simulink model "MPC_stateflow"  (R2018b)
settings: Solver=ode4  StartTime=0.0  StopTime=10  FixedStep=0.05  RelTol=1e-3
libraries: neural x102
(part 3 of 3)

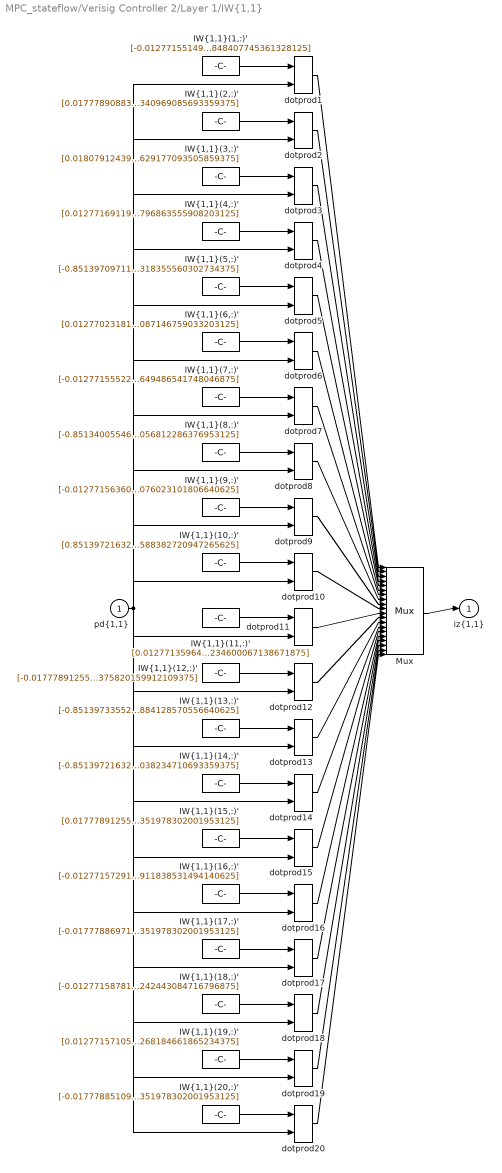
== system MPC_stateflow/Verisig Controller 2/Layer 1/IW{1,1} ==
  "pd{1,1}" : Inport  PortDimensions=6
      mask Display: e = 0.06;c1 = [120 230 180]/255;c2 = ([120 230 180]+0)/(256+128);c3 = ([120 230 180]+128)/(256+128);patch([0 1 1 0],[0 0 1 1],c1);patch([0 1 1 1-e 1-e 0+e],[0 0 1 1-e 0+e 0+e],c2);patch([0 0 1 1-e 0+e 0+e],[0 1 1 1-e 1-e 0+e],c3);plot([0 1 1 0 0],[0 0 1 1 0]);
  "IW{1,1}(1,:)'" : Constant  Value=[-0.012771551497280597686767578125;0.85226726531982421875;0.005031325854361057281494140625;0.0104131400585174560546875;0.52280867099761962890625;0.0038109351880848407745361328125]
      mask Display: e = 0.06;c1 = [120 150 230]/255;c2 = ([120 150 230]+0)/383;c3 = ([120 150 230]+128)/383;patch([0 1 1 0],[0 0 1 1],c1);patch([0 1 1 1-e 1-e 0+e],[0 0 1 1-e 0+e 0+e],c2);patch([0 0 1 1-e 0+e 0+e],[0 1 1 1-e 1-e 0+e],c3);plot([0 1 1 0 0],[0 0 1 1 0]);disp('Weights');
  "IW{1,1}(10,:)'" : Constant  Value=[0.851397216320037841796875;0.016397155821323394775390625;0.01527906768023967742919921875;0.523764669895172119140625;0.0148618109524250030517578125;0.008371211588382720947265625]
      mask Display: e = 0.06;c1 = [120 150 230]/255;c2 = ([120 150 230]+0)/383;c3 = ([120 150 230]+128)/383;patch([0 1 1 0],[0 0 1 1],c1);patch([0 1 1 1-e 1-e 0+e],[0 0 1 1-e 0+e 0+e],c2);patch([0 0 1 1-e 0+e 0+e],[0 1 1 1-e 1-e 0+e],c3);plot([0 1 1 0 0],[0 0 1 1 0]);disp('Weights');
  "IW{1,1}(11,:)'" : Constant  Value=[0.012771359644830226898193359375;-0.85226726531982421875;-0.0050320657901465892791748046875;-0.01041328720748424530029296875;-0.52280867099761962890625;-0.00381127069704234600067138671875]
      mask Display: e = 0.06;c1 = [120 150 230]/255;c2 = ([120 150 230]+0)/383;c3 = ([120 150 230]+128)/383;patch([0 1 1 0],[0 0 1 1],c1);patch([0 1 1 1-e 1-e 0+e],[0 0 1 1-e 0+e 0+e],c2);patch([0 0 1 1-e 0+e 0+e],[0 1 1 1-e 1-e 0+e],c3);plot([0 1 1 0 0],[0 0 1 1 0]);disp('Weights');
  "IW{1,1}(12,:)'" : Constant  Value=[-0.01777891255915164947509765625;-0.011899505741894245147705078125;0.8380184173583984375;-0.010888525284826755523681640625;-0.011424724943935871124267578125;0.54499375820159912109375]
      mask Display: e = 0.06;c1 = [120 150 230]/255;c2 = ([120 150 230]+0)/383;c3 = ([120 150 230]+128)/383;patch([0 1 1 0],[0 0 1 1],c1);patch([0 1 1 1-e 1-e 0+e],[0 0 1 1-e 0+e 0+e],c2);patch([0 0 1 1-e 0+e 0+e],[0 1 1 1-e 1-e 0+e],c3);plot([0 1 1 0 0],[0 0 1 1 0]);disp('Weights');
  "IW{1,1}(13,:)'" : Constant  Value=[-0.851397335529327392578125;-0.01639718003571033477783203125;-0.01527908630669116973876953125;-0.5237643718719482421875;-0.014861813746392726898193359375;-0.00837124884128570556640625]
      mask Display: e = 0.06;c1 = [120 150 230]/255;c2 = ([120 150 230]+0)/383;c3 = ([120 150 230]+128)/383;patch([0 1 1 0],[0 0 1 1],c1);patch([0 1 1 1-e 1-e 0+e],[0 0 1 1-e 0+e 0+e],c2);patch([0 0 1 1-e 0+e 0+e],[0 1 1 1-e 1-e 0+e],c3);plot([0 1 1 0 0],[0 0 1 1 0]);disp('Weights');
  "IW{1,1}(14,:)'" : Constant  Value=[-0.851397216320037841796875;-0.01639718748629093170166015625;-0.015279074199497699737548828125;-0.523764550685882568359375;-0.014861782081425189971923828125;-0.00837126933038234710693359375]
      mask Display: e = 0.06;c1 = [120 150 230]/255;c2 = ([120 150 230]+0)/383;c3 = ([120 150 230]+128)/383;patch([0 1 1 0],[0 0 1 1],c1);patch([0 1 1 1-e 1-e 0+e],[0 0 1 1-e 0+e 0+e],c2);patch([0 0 1 1-e 0+e 0+e],[0 1 1 1-e 1-e 0+e],c3);plot([0 1 1 0 0],[0 0 1 1 0]);disp('Weights');
  "IW{1,1}(15,:)'" : Constant  Value=[0.01777891255915164947509765625;0.011899520643055438995361328125;-0.838018596172332763671875;0.010888495482504367828369140625;0.0114247240126132965087890625;-0.54499351978302001953125]
      mask Display: e = 0.06;c1 = [120 150 230]/255;c2 = ([120 150 230]+0)/383;c3 = ([120 150 230]+128)/383;patch([0 1 1 0],[0 0 1 1],c1);patch([0 1 1 1-e 1-e 0+e],[0 0 1 1-e 0+e 0+e],c2);patch([0 0 1 1-e 0+e 0+e],[0 1 1 1-e 1-e 0+e],c3);plot([0 1 1 0 0],[0 0 1 1 0]);disp('Weights');
  "IW{1,1}(16,:)'" : Constant  Value=[-0.0127715729176998138427734375;0.85226726531982421875;0.0050313179381191730499267578125;0.010413181968033313751220703125;0.52280867099761962890625;0.0038109519518911838531494140625]
      mask Display: e = 0.06;c1 = [120 150 230]/255;c2 = ([120 150 230]+0)/383;c3 = ([120 150 230]+128)/383;patch([0 1 1 0],[0 0 1 1],c1);patch([0 1 1 1-e 1-e 0+e],[0 0 1 1-e 0+e 0+e],c2);patch([0 0 1 1-e 0+e 0+e],[0 1 1 1-e 1-e 0+e],c3);plot([0 1 1 0 0],[0 0 1 1 0]);disp('Weights');
  "IW{1,1}(17,:)'" : Constant  Value=[-0.0177788697183132171630859375;-0.01189949549734592437744140625;0.83801853656768798828125;-0.010888428427278995513916015625;-0.011424727737903594970703125;0.54499351978302001953125]
      mask Display: e = 0.06;c1 = [120 150 230]/255;c2 = ([120 150 230]+0)/383;c3 = ([120 150 230]+128)/383;patch([0 1 1 0],[0 0 1 1],c1);patch([0 1 1 1-e 1-e 0+e],[0 0 1 1-e 0+e 0+e],c2);patch([0 0 1 1-e 0+e 0+e],[0 1 1 1-e 1-e 0+e],c3);plot([0 1 1 0 0],[0 0 1 1 0]);disp('Weights');
  "IW{1,1}(18,:)'" : Constant  Value=[-0.0127715878188610076904296875;0.852267444133758544921875;0.0050312615931034088134765625;0.010413181968033313751220703125;0.52280843257904052734375;0.00381095963530242443084716796875]
      mask Display: e = 0.06;c1 = [120 150 230]/255;c2 = ([120 150 230]+0)/383;c3 = ([120 150 230]+128)/383;patch([0 1 1 0],[0 0 1 1],c1);patch([0 1 1 1-e 1-e 0+e],[0 0 1 1-e 0+e 0+e],c2);patch([0 0 1 1-e 0+e 0+e],[0 1 1 1-e 1-e 0+e],c3);plot([0 1 1 0 0],[0 0 1 1 0]);disp('Weights');
  "IW{1,1}(19,:)'" : Constant  Value=[0.01277157105505466461181640625;-0.852267205715179443359375;-0.005031269975006580352783203125;-0.0104131735861301422119140625;-0.522808611392974853515625;-0.0038109286688268184661865234375]
      mask Display: e = 0.06;c1 = [120 150 230]/255;c2 = ([120 150 230]+0)/383;c3 = ([120 150 230]+128)/383;patch([0 1 1 0],[0 0 1 1],c1);patch([0 1 1 1-e 1-e 0+e],[0 0 1 1-e 0+e 0+e],c2);patch([0 0 1 1-e 0+e 0+e],[0 1 1 1-e 1-e 0+e],c3);plot([0 1 1 0 0],[0 0 1 1 0]);disp('Weights');
  "IW{1,1}(2,:)'" : Constant  Value=[0.01777890883386135101318359375;0.011899493634700775146484375;-0.838018715381622314453125;0.01088852994143962860107421875;0.011424682103097438812255859375;-0.544993340969085693359375]
      mask Display: e = 0.06;c1 = [120 150 230]/255;c2 = ([120 150 230]+0)/383;c3 = ([120 150 230]+128)/383;patch([0 1 1 0],[0 0 1 1],c1);patch([0 1 1 1-e 1-e 0+e],[0 0 1 1-e 0+e 0+e],c2);patch([0 0 1 1-e 0+e 0+e],[0 1 1 1-e 1-e 0+e],c3);plot([0 1 1 0 0],[0 0 1 1 0]);disp('Weights');
  "IW{1,1}(20,:)'" : Constant  Value=[-0.017778851091861724853515625;-0.011899485252797603607177734375;0.83801853656768798828125;-0.010888493619859218597412109375;-0.0114247165620326995849609375;0.54499351978302001953125]
      mask Display: e = 0.06;c1 = [120 150 230]/255;c2 = ([120 150 230]+0)/383;c3 = ([120 150 230]+128)/383;patch([0 1 1 0],[0 0 1 1],c1);patch([0 1 1 1-e 1-e 0+e],[0 0 1 1-e 0+e 0+e],c2);patch([0 0 1 1-e 0+e 0+e],[0 1 1 1-e 1-e 0+e],c3);plot([0 1 1 0 0],[0 0 1 1 0]);disp('Weights');
  "IW{1,1}(3,:)'" : Constant  Value=[0.018079124391078948974609375;0.012226282618939876556396484375;-0.8379306793212890625;0.011077952571213245391845703125;0.011494635604321956634521484375;-0.54510629177093505859375]
      mask Display: e = 0.06;c1 = [120 150 230]/255;c2 = ([120 150 230]+0)/383;c3 = ([120 150 230]+128)/383;patch([0 1 1 0],[0 0 1 1],c1);patch([0 1 1 1-e 1-e 0+e],[0 0 1 1-e 0+e 0+e],c2);patch([0 0 1 1-e 0+e 0+e],[0 1 1 1-e 1-e 0+e],c3);plot([0 1 1 0 0],[0 0 1 1 0]);disp('Weights');
  "IW{1,1}(4,:)'" : Constant  Value=[0.012771691195666790008544921875;-0.852267205715179443359375;-0.005030765198171138763427734375;-0.010413102805614471435546875;-0.5228087902069091796875;-0.00381070119328796863555908203125]
      mask Display: e = 0.06;c1 = [120 150 230]/255;c2 = ([120 150 230]+0)/383;c3 = ([120 150 230]+128)/383;patch([0 1 1 0],[0 0 1 1],c1);patch([0 1 1 1-e 1-e 0+e],[0 0 1 1-e 0+e 0+e],c2);patch([0 0 1 1-e 0+e 0+e],[0 1 1 1-e 1-e 0+e],c3);plot([0 1 1 0 0],[0 0 1 1 0]);disp('Weights');
  "IW{1,1}(5,:)'" : Constant  Value=[-0.851397097110748291015625;-0.01639718748629093170166015625;-0.015279111452400684356689453125;-0.52376461029052734375;-0.014861795119941234588623046875;-0.008371188305318355560302734375]
      mask Display: e = 0.06;c1 = [120 150 230]/255;c2 = ([120 150 230]+0)/383;c3 = ([120 150 230]+128)/383;patch([0 1 1 0],[0 0 1 1],c1);patch([0 1 1 1-e 1-e 0+e],[0 0 1 1-e 0+e 0+e],c2);patch([0 0 1 1-e 0+e 0+e],[0 1 1 1-e 1-e 0+e],c3);plot([0 1 1 0 0],[0 0 1 1 0]);disp('Weights');
  "IW{1,1}(6,:)'" : Constant  Value=[0.0127702318131923675537109375;-0.852267563343048095703125;-0.0050366655923426151275634765625;-0.010414107702672481536865234375;-0.522808074951171875;-0.003813070245087146759033203125]
      mask Display: e = 0.06;c1 = [120 150 230]/255;c2 = ([120 150 230]+0)/383;c3 = ([120 150 230]+128)/383;patch([0 1 1 0],[0 0 1 1],c1);patch([0 1 1 1-e 1-e 0+e],[0 0 1 1-e 0+e 0+e],c2);patch([0 0 1 1-e 0+e 0+e],[0 1 1 1-e 1-e 0+e],c3);plot([0 1 1 0 0],[0 0 1 1 0]);disp('Weights');
  "IW{1,1}(7,:)'" : Constant  Value=[-0.012771555222570896148681640625;0.85226726531982421875;0.0050313002429902553558349609375;0.01041315495967864990234375;0.52280867099761962890625;0.003810915164649486541748046875]
      mask Display: e = 0.06;c1 = [120 150 230]/255;c2 = ([120 150 230]+0)/383;c3 = ([120 150 230]+128)/383;patch([0 1 1 0],[0 0 1 1],c1);patch([0 1 1 1-e 1-e 0+e],[0 0 1 1-e 0+e 0+e],c2);patch([0 0 1 1-e 0+e 0+e],[0 1 1 1-e 1-e 0+e],c3);plot([0 1 1 0 0],[0 0 1 1 0]);disp('Weights');
  "IW{1,1}(8,:)'" : Constant  Value=[-0.8513400554656982421875;-0.017523847520351409912109375;-0.01597718894481658935546875;-0.523753225803375244140625;-0.015967547893524169921875;-0.009223726578056812286376953125]
      mask Display: e = 0.06;c1 = [120 150 230]/255;c2 = ([120 150 230]+0)/383;c3 = ([120 150 230]+128)/383;patch([0 1 1 0],[0 0 1 1],c1);patch([0 1 1 1-e 1-e 0+e],[0 0 1 1-e 0+e 0+e],c2);patch([0 0 1 1-e 0+e 0+e],[0 1 1 1-e 1-e 0+e],c3);plot([0 1 1 0 0],[0 0 1 1 0]);disp('Weights');
  "IW{1,1}(9,:)'" : Constant  Value=[-0.01277156360447406768798828125;0.852267205715179443359375;0.0050313319079577922821044921875;0.010413155891001224517822265625;0.5228087902069091796875;0.0038109072484076023101806640625]
      mask Display: e = 0.06;c1 = [120 150 230]/255;c2 = ([120 150 230]+0)/383;c3 = ([120 150 230]+128)/383;patch([0 1 1 0],[0 0 1 1],c1);patch([0 1 1 1-e 1-e 0+e],[0 0 1 1-e 0+e 0+e],c2);patch([0 0 1 1-e 0+e 0+e],[0 1 1 1-e 1-e 0+e],c3);plot([0 1 1 0 0],[0 0 1 1 0]);disp('Weights');
  Mux : Mux  Inputs=20
      mask Display: e = 0.06;c1 = [120 150 230]/255;c2 = ([120 150 230]+0)/383;c3 = ([120 150 230]+128)/383;patch([0 1 1 0],[0 0 1 1],c1);patch([0 1 1 1-e 1-e 0+e],[0 0 1 1-e 0+e 0+e],c2);patch([0 0 1 1-e 0+e 0+e],[0 1 1 1-e 1-e 0+e],c3);plot([0 1 1 0 0],[0 0 1 1 0]);disp('Mux');
  dotprod{1..20} (20 alike) : neural/Weight Functions/dotprod
  "iz{1,1}" : Outport
      mask Display: e = 0.06;c1 = [120 230 180]/255;c2 = ([120 230 180]+0)/(256+128);c3 = ([120 230 180]+128)/(256+128);patch([0 1 1 0],[0 0 1 1],c1);patch([0 1 1 1-e 1-e 0+e],[0 0 1 1-e 0+e 0+e],c2);patch([0 0 1 1-e 0+e 0+e],[0 1 1 1-e 1-e 0+e],c3);plot([0 1 1 0 0],[0 0 1 1 0]);
  wires:
  Mux/1 -> "iz{1,1}"/1
  dotprod20/1 -> Mux/20
  "IW{1,1}(20,:)'"/1 -> dotprod20/1
  dotprod19/1 -> Mux/19
  "IW{1,1}(19,:)'"/1 -> dotprod19/1
  dotprod18/1 -> Mux/18
  "IW{1,1}(18,:)'"/1 -> dotprod18/1
  dotprod17/1 -> Mux/17
  "IW{1,1}(17,:)'"/1 -> dotprod17/1
  dotprod16/1 -> Mux/16
  "IW{1,1}(16,:)'"/1 -> dotprod16/1
  dotprod15/1 -> Mux/15
  "IW{1,1}(15,:)'"/1 -> dotprod15/1
  dotprod14/1 -> Mux/14
  "IW{1,1}(14,:)'"/1 -> dotprod14/1
  dotprod13/1 -> Mux/13
  "IW{1,1}(13,:)'"/1 -> dotprod13/1
  dotprod12/1 -> Mux/12
  "IW{1,1}(12,:)'"/1 -> dotprod12/1
  dotprod11/1 -> Mux/11
  "IW{1,1}(11,:)'"/1 -> dotprod11/1
  dotprod10/1 -> Mux/10
  "IW{1,1}(10,:)'"/1 -> dotprod10/1
  dotprod9/1 -> Mux/9
  "IW{1,1}(9,:)'"/1 -> dotprod9/1
  dotprod8/1 -> Mux/8
  "IW{1,1}(8,:)'"/1 -> dotprod8/1
  dotprod7/1 -> Mux/7
  "IW{1,1}(7,:)'"/1 -> dotprod7/1
  dotprod6/1 -> Mux/6
  "IW{1,1}(6,:)'"/1 -> dotprod6/1
  dotprod5/1 -> Mux/5
  "IW{1,1}(5,:)'"/1 -> dotprod5/1
  dotprod4/1 -> Mux/4
  "IW{1,1}(4,:)'"/1 -> dotprod4/1
  dotprod3/1 -> Mux/3
  "IW{1,1}(3,:)'"/1 -> dotprod3/1
  dotprod2/1 -> Mux/2
  "IW{1,1}(2,:)'"/1 -> dotprod2/1
  dotprod1/1 -> Mux/1
  "pd{1,1}"/1 -> dotprod20/2, dotprod19/2, dotprod18/2, dotprod17/2, dotprod16/2, dotprod15/2, dotprod14/2, dotprod13/2, dotprod12/2, dotprod11/2, dotprod10/2, dotprod9/2, dotprod8/2, dotprod7/2, dotprod6/2, dotprod5/2, dotprod4/2, dotprod3/2, dotprod2/2, dotprod1/2
  "IW{1,1}(1,:)'"/1 -> dotprod1/1

== system MPC_stateflow/Verisig Controller 2/Layer 2/Delays 1 ==
  "p{2}" : Inport  PortDimensions=20
      mask Display: e = 0.06;c1 = [120 230 180]/255;c2 = ([120 230 180]+0)/(256+128);c3 = ([120 230 180]+128)/(256+128);patch([0 1 1 0],[0 0 1 1],c1);patch([0 1 1 1-e 1-e 0+e],[0 0 1 1-e 0+e 0+e],c2);patch([0 0 1 1-e 0+e 0+e],[0 1 1 1-e 1-e 0+e],c3);plot([0 1 1 0 0],[0 0 1 1 0]);
  mux : Mux  Inputs=1
      mask Display: e = 0.06;c1 = [120 150 230]/255;c2 = ([120 150 230]+0)/383;c3 = ([120 150 230]+128)/383;patch([0 1 1 0],[0 0 1 1],c1);patch([0 1 1 1-e 1-e 0+e],[0 0 1 1-e 0+e 0+e],c2);patch([0 0 1 1-e 0+e 0+e],[0 1 1 1-e 1-e 0+e],c3);plot([0 1 1 0 0],[0 0 1 1 0]);disp('Mux')
  "pd{2,1}" : Outport
      mask Display: e = 0.06;c1 = [120 230 180]/255;c2 = ([120 230 180]+0)/(256+128);c3 = ([120 230 180]+128)/(256+128);patch([0 1 1 0],[0 0 1 1],c1);patch([0 1 1 1-e 1-e 0+e],[0 0 1 1-e 0+e 0+e],c2);patch([0 0 1 1-e 0+e 0+e],[0 1 1 1-e 1-e 0+e],c3);plot([0 1 1 0 0],[0 0 1 1 0]);
  wires:
  mux/1 -> "pd{2,1}"/1
  "p{2}"/1 -> mux/1

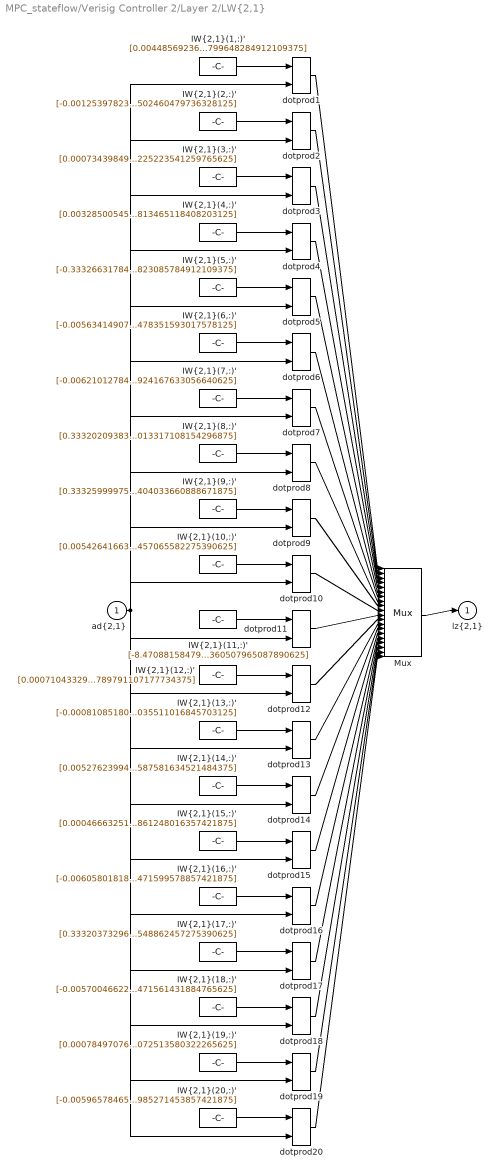
== system MPC_stateflow/Verisig Controller 2/Layer 2/LW{2,1} ==
  "ad{2,1}" : Inport  PortDimensions=20
      mask Display: e = 0.06;c1 = [120 230 180]/255;c2 = ([120 230 180]+0)/(256+128);c3 = ([120 230 180]+128)/(256+128);patch([0 1 1 0],[0 0 1 1],c1);patch([0 1 1 1-e 1-e 0+e],[0 0 1 1-e 0+e 0+e],c2);patch([0 0 1 1-e 0+e 0+e],[0 1 1 1-e 1-e 0+e],c3);plot([0 1 1 0 0],[0 0 1 1 0]);
  "IW{2,1}(1,:)'" : Constant  Value=[0.0044856923632323741912841796875;0.4092908799648284912109375;0.402330338954925537109375;-0.0044856867752969264984130859375;-0.0084942989051342010498046875;-0.0044855973683297634124755859375;0.00448568724095821380615234375;-0.008073708973824977874755859375;0.004485689103603363037109375;0.0084942989051342010498046875;-0.004485669545829296112060546875;-0.40929090976715087890625;-0.008494290523231029510498046875;-0.0084942914545536041259765625;0.4092908799648284912109375;0.0044856821186840534210205078125;-0.4092908799648284912109375;0.0044856853783130645751953125;-0.00448568351566791534423828125;-0.4092908799648284912109375]
      mask Display: e = 0.06;c1 = [120 150 230]/255;c2 = ([120 150 230]+0)/383;c3 = ([120 150 230]+128)/383;patch([0 1 1 0],[0 0 1 1],c1);patch([0 1 1 1-e 1-e 0+e],[0 0 1 1-e 0+e 0+e],c2);patch([0 0 1 1-e 0+e 0+e],[0 1 1 1-e 1-e 0+e],c3);plot([0 1 1 0 0],[0 0 1 1 0]);disp('weights');
  "IW{2,1}(10,:)'" : Constant  Value=[0.0054264166392385959625244140625;0.012804088182747364044189453125;0.012594926171004772186279296875;-0.0054266476072371006011962890625;-0.4481963217258453369140625;-0.0054238340817391872406005859375;0.0054264296777546405792236328125;-0.4418563544750213623046875;0.0054264222271740436553955078125;0.448196232318878173828125;-0.0054260306060314178466796875;-0.012804095633327960968017578125;-0.448196232318878173828125;-0.4481961727142333984375;0.012804099358618259429931640625;0.0054264306090772151947021484375;-0.012804084457457065582275390625;0.0054264315403997898101806640625;-0.005426420830190181732177734375;-0.012804084457457065582275390625]
      mask Display: e = 0.06;c1 = [120 150 230]/255;c2 = ([120 150 230]+0)/383;c3 = ([120 150 230]+128)/383;patch([0 1 1 0],[0 0 1 1],c1);patch([0 1 1 1-e 1-e 0+e],[0 0 1 1-e 0+e 0+e],c2);patch([0 0 1 1-e 0+e 0+e],[0 1 1 1-e 1-e 0+e],c3);plot([0 1 1 0 0],[0 0 1 1 0]);disp('weights');
  "IW{2,1}(11,:)'" : Constant  Value=[-8.47088158479891717433929443359375e-05;-0.01166805811226367950439453125;-0.011431642808020114898681640625;8.49300486152060329914093017578125e-05;0.4482459723949432373046875;8.2065365859307348728179931640625e-05;-8.470812463201582431793212890625e-05;0.442142784595489501953125;-8.47004484967328608036041259765625e-05;-0.448246002197265625;8.4288840298540890216827392578125e-05;0.0116680599749088287353515625;0.448246002197265625;0.4482459723949432373046875;-0.01166805066168308258056640625;-8.47076225909404456615447998046875e-05;0.011668048799037933349609375;-8.4695915575139224529266357421875e-05;8.47055925987660884857177734375e-05;0.011668049730360507965087890625]
      mask Display: e = 0.06;c1 = [120 150 230]/255;c2 = ([120 150 230]+0)/383;c3 = ([120 150 230]+128)/383;patch([0 1 1 0],[0 0 1 1],c1);patch([0 1 1 1-e 1-e 0+e],[0 0 1 1-e 0+e 0+e],c2);patch([0 0 1 1-e 0+e 0+e],[0 1 1 1-e 1-e 0+e],c3);plot([0 1 1 0 0],[0 0 1 1 0]);disp('weights');
  "IW{2,1}(12,:)'" : Constant  Value=[0.0007104332908056676387786865234375;-0.0121032260358333587646484375;-0.011863806284964084625244140625;-0.0007102005183696746826171875;0.448233664035797119140625;-0.00071304966695606708526611328125;0.000710433465428650379180908203125;0.44211804866790771484375;0.0007104235119186341762542724609375;-0.4482336342334747314453125;-0.00071082473732531070709228515625;0.01210323907434940338134765625;0.4482337534427642822265625;0.4482335746288299560546875;-0.012103230692446231842041015625;0.0007104267715476453304290771484375;0.01210322044789791107177734375;0.00071042799390852451324462890625;-0.0007104240357875823974609375;0.01210322044789791107177734375]
      mask Display: e = 0.06;c1 = [120 150 230]/255;c2 = ([120 150 230]+0)/383;c3 = ([120 150 230]+128)/383;patch([0 1 1 0],[0 0 1 1],c1);patch([0 1 1 1-e 1-e 0+e],[0 0 1 1-e 0+e 0+e],c2);patch([0 0 1 1-e 0+e 0+e],[0 1 1 1-e 1-e 0+e],c3);plot([0 1 1 0 0],[0 0 1 1 0]);disp('weights');
  "IW{2,1}(13,:)'" : Constant  Value=[-0.0008108518086373805999755859375;-0.011628665030002593994140625;-0.011395211331546306610107421875;0.00081110117025673389434814453125;0.4482516348361968994140625;0.000808243756182491779327392578125;-0.0008108714246191084384918212890625;0.442119419574737548828125;-0.0008108730544336140155792236328125;-0.44825160503387451171875;0.0008104708977043628692626953125;0.01162867248058319091796875;0.44825160503387451171875;0.4482516348361968994140625;-0.0116286613047122955322265625;-0.0008108695619739592075347900390625;0.0116286464035511016845703125;-0.0008108615875244140625;0.0008108713664114475250244140625;0.0116286464035511016845703125]
      mask Display: e = 0.06;c1 = [120 150 230]/255;c2 = ([120 150 230]+0)/383;c3 = ([120 150 230]+128)/383;patch([0 1 1 0],[0 0 1 1],c1);patch([0 1 1 1-e 1-e 0+e],[0 0 1 1-e 0+e 0+e],c2);patch([0 0 1 1-e 0+e 0+e],[0 1 1 1-e 1-e 0+e],c3);plot([0 1 1 0 0],[0 0 1 1 0]);disp('weights');
  "IW{2,1}(14,:)'" : Constant  Value=[0.0052762399427592754364013671875;0.4092657268047332763671875;0.402362406253814697265625;-0.00527626089751720428466796875;-0.008586729876697063446044921875;-0.0052761598490178585052490234375;0.0052762380801141262054443359375;-0.00816504098474979400634765625;0.0052762464620172977447509765625;0.008586726151406764984130859375;-0.005276233889162540435791015625;-0.409265697002410888671875;-0.00858672522008419036865234375;-0.00858671776950359344482421875;0.409265697002410888671875;0.0052762539125978946685791015625;-0.4092657566070556640625;0.00527624972164630889892578125;-0.0052762539125978946685791015625;-0.40926587581634521484375]
      mask Display: e = 0.06;c1 = [120 150 230]/255;c2 = ([120 150 230]+0)/383;c3 = ([120 150 230]+128)/383;patch([0 1 1 0],[0 0 1 1],c1);patch([0 1 1 1-e 1-e 0+e],[0 0 1 1-e 0+e 0+e],c2);patch([0 0 1 1-e 0+e 0+e],[0 1 1 1-e 1-e 0+e],c3);plot([0 1 1 0 0],[0 0 1 1 0]);disp('weights');
  "IW{2,1}(15,:)'" : Constant  Value=[0.00046663251123391091823577880859375;-0.0120042599737644195556640625;-0.011765711009502410888671875;-0.0004664020962081849575042724609375;0.448237001895904541015625;-0.000469259801320731639862060546875;0.0004666281747631728649139404296875;0.4421238601207733154296875;0.0004666206077672541141510009765625;-0.448236882686614990234375;-0.00046703135012648999691009521484375;0.012004264630377292633056640625;0.448236942291259765625;0.44823682308197021484375;-0.01200425811111927032470703125;0.00046662942622788250446319580078125;0.012004253454506397247314453125;0.0004666416789405047893524169921875;-0.00046663961256854236125946044921875;0.012004251591861248016357421875]
      mask Display: e = 0.06;c1 = [120 150 230]/255;c2 = ([120 150 230]+0)/383;c3 = ([120 150 230]+128)/383;patch([0 1 1 0],[0 0 1 1],c1);patch([0 1 1 1-e 1-e 0+e],[0 0 1 1-e 0+e 0+e],c2);patch([0 0 1 1-e 0+e 0+e],[0 1 1 1-e 1-e 0+e],c3);plot([0 1 1 0 0],[0 0 1 1 0]);disp('weights');
  "IW{2,1}(16,:)'" : Constant  Value=[-0.0060580181889235973358154296875;-0.4092471599578857421875;-0.402382314205169677734375;0.006058032624423503875732421875;0.00835076160728931427001953125;0.0060579092241823673248291015625;-0.00605802051723003387451171875;0.0079286098480224609375;-0.0060580228455364704132080078125;-0.0083507709205150604248046875;0.0060580060817301273345947265625;0.4092471897602081298828125;0.0083507709205150604248046875;0.0083507709205150604248046875;-0.4092471599578857421875;-0.00605802237987518310546875;0.409247219562530517578125;-0.0060580135323107242584228515625;0.006058021448552608489990234375;0.4092471599578857421875]
      mask Display: e = 0.06;c1 = [120 150 230]/255;c2 = ([120 150 230]+0)/383;c3 = ([120 150 230]+128)/383;patch([0 1 1 0],[0 0 1 1],c1);patch([0 1 1 1-e 1-e 0+e],[0 0 1 1-e 0+e 0+e],c2);patch([0 0 1 1-e 0+e 0+e],[0 1 1 1-e 1-e 0+e],c3);plot([0 1 1 0 0],[0 0 1 1 0]);disp('weights');
  "IW{2,1}(17,:)'" : Constant  Value=[0.333203732967376708984375;0.00331465131603181362152099609375;0.0033306344412267208099365234375;-0.3332033455371856689453125;-0.01178176514804363250732421875;-0.333208143711090087890625;0.333203613758087158203125;-0.012370237149298191070556640625;0.3332037031650543212890625;0.01178176701068878173828125;-0.33320438861846923828125;-0.00331464991904795169830322265625;-0.011781766079366207122802734375;-0.01178176701068878173828125;0.00331465783528983592987060546875;0.333203732967376708984375;-0.00331465597264468669891357421875;0.33320367336273193359375;-0.333203732967376708984375;-0.003314651548862457275390625]
      mask Display: e = 0.06;c1 = [120 150 230]/255;c2 = ([120 150 230]+0)/383;c3 = ([120 150 230]+128)/383;patch([0 1 1 0],[0 0 1 1],c1);patch([0 1 1 1-e 1-e 0+e],[0 0 1 1-e 0+e 0+e],c2);patch([0 0 1 1-e 0+e 0+e],[0 1 1 1-e 1-e 0+e],c3);plot([0 1 1 0 0],[0 0 1 1 0]);disp('weights');
  "IW{2,1}(18,:)'" : Constant  Value=[-0.005700466223061084747314453125;-0.4092574417591094970703125;-0.4023625552654266357421875;0.0057004974223673343658447265625;0.0084886066615581512451171875;0.005700360052287578582763671875;-0.0057004666887223720550537109375;0.00806747935712337493896484375;-0.005700477398931980133056640625;-0.0084886141121387481689453125;0.005700456909835338592529296875;0.4092574417591094970703125;0.008488607592880725860595703125;0.008488602004945278167724609375;-0.4092575013637542724609375;-0.005700466223061084747314453125;0.4092575013637542724609375;-0.0057004629634320735931396484375;0.00570046901702880859375;0.409257471561431884765625]
      mask Display: e = 0.06;c1 = [120 150 230]/255;c2 = ([120 150 230]+0)/383;c3 = ([120 150 230]+128)/383;patch([0 1 1 0],[0 0 1 1],c1);patch([0 1 1 1-e 1-e 0+e],[0 0 1 1-e 0+e 0+e],c2);patch([0 0 1 1-e 0+e 0+e],[0 1 1 1-e 1-e 0+e],c3);plot([0 1 1 0 0],[0 0 1 1 0]);disp('weights');
  "IW{2,1}(19,:)'" : Constant  Value=[0.0007849707617424428462982177734375;0.0121510140597820281982421875;0.011918344534933567047119140625;-0.0007852140697650611400604248046875;-0.4482424557209014892578125;-0.0007823808700777590274810791015625;0.0007849783287383615970611572265625;-0.442073285579681396484375;0.0007849846151657402515411376953125;0.4482424259185791015625;-0.0007845927611924707889556884765625;-0.012151009403169155120849609375;-0.4482423961162567138671875;-0.4482423961162567138671875;0.012150995433330535888671875;0.0007849778048694133758544921875;-0.012150992639362812042236328125;0.0007849839166738092899322509765625;-0.0007849822868593037128448486328125;-0.012150988914072513580322265625]
      mask Display: e = 0.06;c1 = [120 150 230]/255;c2 = ([120 150 230]+0)/383;c3 = ([120 150 230]+128)/383;patch([0 1 1 0],[0 0 1 1],c1);patch([0 1 1 1-e 1-e 0+e],[0 0 1 1-e 0+e 0+e],c2);patch([0 0 1 1-e 0+e 0+e],[0 1 1 1-e 1-e 0+e],c3);plot([0 1 1 0 0],[0 0 1 1 0]);disp('weights');
  "IW{2,1}(2,:)'" : Constant  Value=[-0.001253978232853114604949951171875;0.011227603070437908172607421875;0.010983745567500591278076171875;0.00125373830087482929229736328125;-0.448236286640167236328125;0.0012566098012030124664306640625;-0.001253973809070885181427001953125;-0.44223487377166748046875;-0.001253968919627368450164794921875;0.4482362568378448486328125;0.0012543690390884876251220703125;-0.011227612383663654327392578125;-0.4482363164424896240234375;-0.448236167430877685546875;0.011227606795728206634521484375;-0.001253972644917666912078857421875;-0.011227593757212162017822265625;-0.00125397532247006893157958984375;0.0012539732269942760467529296875;-0.011227597482502460479736328125]
      mask Display: e = 0.06;c1 = [120 150 230]/255;c2 = ([120 150 230]+0)/383;c3 = ([120 150 230]+128)/383;patch([0 1 1 0],[0 0 1 1],c1);patch([0 1 1 1-e 1-e 0+e],[0 0 1 1-e 0+e 0+e],c2);patch([0 0 1 1-e 0+e 0+e],[0 1 1 1-e 1-e 0+e],c3);plot([0 1 1 0 0],[0 0 1 1 0]);disp('weights');
  "IW{2,1}(20,:)'" : Constant  Value=[-0.0059657846577465534210205078125;-0.4092517793178558349609375;-0.402370870113372802734375;0.005965803749859333038330078125;0.00834904797375202178955078125;0.0059656738303601741790771484375;-0.0059657874517142772674560546875;0.00792670063674449920654296875;-0.00596578232944011688232421875;-0.008349056355655193328857421875;0.00596577115356922149658203125;0.40925180912017822265625;0.008349052630364894866943359375;0.00834904052317142486572265625;-0.40925180912017822265625;-0.005965786986052989959716796875;0.4092519581317901611328125;-0.005965786986052989959716796875;0.0059657902456820011138916015625;0.4092518985271453857421875]
      mask Display: e = 0.06;c1 = [120 150 230]/255;c2 = ([120 150 230]+0)/383;c3 = ([120 150 230]+128)/383;patch([0 1 1 0],[0 0 1 1],c1);patch([0 1 1 1-e 1-e 0+e],[0 0 1 1-e 0+e 0+e],c2);patch([0 0 1 1-e 0+e 0+e],[0 1 1 1-e 1-e 0+e],c3);plot([0 1 1 0 0],[0 0 1 1 0]);disp('weights');
  "IW{2,1}(3,:)'" : Constant  Value=[0.000734398490749299526214599609375;-0.011749573983252048492431640625;-0.011509227566421031951904296875;-0.00073416717350482940673828125;0.448237240314483642578125;-0.0007370298844762146472930908203125;0.00073438300751149654388427734375;0.4421602189540863037109375;0.0007343870238400995731353759765625;-0.4482371807098388671875;-0.0007348008803091943264007568359375;0.011749575845897197723388671875;0.448237240314483642578125;0.4482372105121612548828125;-0.0117495693266391754150390625;0.000734380329959094524383544921875;0.01174954883754253387451171875;0.0007343843462876975536346435546875;-0.000734395231120288372039794921875;0.01174954511225223541259765625]
      mask Display: e = 0.06;c1 = [120 150 230]/255;c2 = ([120 150 230]+0)/383;c3 = ([120 150 230]+128)/383;patch([0 1 1 0],[0 0 1 1],c1);patch([0 1 1 1-e 1-e 0+e],[0 0 1 1-e 0+e 0+e],c2);patch([0 0 1 1-e 0+e 0+e],[0 1 1 1-e 1-e 0+e],c3);plot([0 1 1 0 0],[0 0 1 1 0]);disp('weights');
  "IW{2,1}(4,:)'" : Constant  Value=[0.00328500545583665370941162109375;0.012248189188539981842041015625;0.0120280645787715911865234375;-0.003285229206085205078125;-0.4482342302799224853515625;-0.0032824152149260044097900390625;0.003285015933215618133544921875;-0.4419864714145660400390625;0.00328501383773982524871826171875;0.4482343196868896484375;-0.003284617327153682708740234375;-0.01224819384515285491943359375;-0.44823420047760009765625;-0.448234260082244873046875;0.012248180806636810302734375;0.00328501290641725063323974609375;-0.012248178012669086456298828125;0.0032850126735866069793701171875;-0.00328501057811081409454345703125;-0.0122481770813465118408203125]
      mask Display: e = 0.06;c1 = [120 150 230]/255;c2 = ([120 150 230]+0)/383;c3 = ([120 150 230]+128)/383;patch([0 1 1 0],[0 0 1 1],c1);patch([0 1 1 1-e 1-e 0+e],[0 0 1 1-e 0+e 0+e],c2);patch([0 0 1 1-e 0+e 0+e],[0 1 1 1-e 1-e 0+e],c3);plot([0 1 1 0 0],[0 0 1 1 0]);disp('weights');
  "IW{2,1}(5,:)'" : Constant  Value=[-0.333266317844390869140625;0.00128670991398394107818603515625;0.001274360693059861660003662109375;0.333266317844390869140625;0.008707520551979541778564453125;0.3332684338092803955078125;-0.3332663476467132568359375;0.009328183718025684356689453125;-0.3332663476467132568359375;-0.0087075270712375640869140625;0.3332668244838714599609375;-0.001286706537939608097076416015625;0.008707529865205287933349609375;0.00870752893388271331787109375;0.0012867064215242862701416015625;-0.3332663476467132568359375;-0.00128669920377433300018310546875;-0.33326625823974609375;0.3332662880420684814453125;-0.0012867129407823085784912109375]
      mask Display: e = 0.06;c1 = [120 150 230]/255;c2 = ([120 150 230]+0)/383;c3 = ([120 150 230]+128)/383;patch([0 1 1 0],[0 0 1 1],c1);patch([0 1 1 1-e 1-e 0+e],[0 0 1 1-e 0+e 0+e],c2);patch([0 0 1 1-e 0+e 0+e],[0 1 1 1-e 1-e 0+e],c3);plot([0 1 1 0 0],[0 0 1 1 0]);disp('weights');
  "IW{2,1}(6,:)'" : Constant  Value=[-0.0056341490708291530609130859375;-0.4092621505260467529296875;-0.4023561179637908935546875;0.005634183995425701141357421875;0.008391384966671466827392578125;0.0056340550072491168975830078125;-0.005634150467813014984130859375;0.0079695247113704681396484375;-0.005634148605167865753173828125;-0.00839138589799404144287109375;0.0056341500021517276763916015625;0.409262239933013916015625;0.008391381241381168365478515625;0.00839137472212314605712890625;-0.4092624485492706298828125;-0.0056341588497161865234375;0.4092624485492706298828125;-0.005634146742522716522216796875;0.0056341462768614292144775390625;0.409262478351593017578125]
      mask Display: e = 0.06;c1 = [120 150 230]/255;c2 = ([120 150 230]+0)/383;c3 = ([120 150 230]+128)/383;patch([0 1 1 0],[0 0 1 1],c1);patch([0 1 1 1-e 1-e 0+e],[0 0 1 1-e 0+e 0+e],c2);patch([0 0 1 1-e 0+e 0+e],[0 1 1 1-e 1-e 0+e],c3);plot([0 1 1 0 0],[0 0 1 1 0]);disp('weights');
  "IW{2,1}(7,:)'" : Constant  Value=[-0.00621012784540653228759765625;-0.40924167633056640625;-0.402368247509002685546875;0.006210171617567539215087890625;0.0085550211369991302490234375;0.00621003098785877227783203125;-0.0062101292423903942108154296875;0.008134675212204456329345703125;-0.0062101320363581180572509765625;-0.008555027656257152557373046875;0.00621012039482593536376953125;0.40924167633056640625;0.00855500809848308563232421875;0.0085550136864185333251953125;-0.40924167633056640625;-0.0062101255171000957489013671875;0.4092416465282440185546875;-0.0062101283110678195953369140625;0.006210136227309703826904296875;0.40924167633056640625]
      mask Display: e = 0.06;c1 = [120 150 230]/255;c2 = ([120 150 230]+0)/383;c3 = ([120 150 230]+128)/383;patch([0 1 1 0],[0 0 1 1],c1);patch([0 1 1 1-e 1-e 0+e],[0 0 1 1-e 0+e 0+e],c2);patch([0 0 1 1-e 0+e 0+e],[0 1 1 1-e 1-e 0+e],c3);plot([0 1 1 0 0],[0 0 1 1 0]);disp('weights');
  "IW{2,1}(8,:)'" : Constant  Value=[0.3332020938396453857421875;0.0034835836850106716156005859375;0.003498683683574199676513671875;-0.3332015573978424072265625;-0.01180832646787166595458984375;-0.3332063853740692138671875;0.3332020342350006103515625;-0.01239728741347789764404296875;0.3332020342350006103515625;0.011808327399194240570068359375;-0.333202779293060302734375;-0.00348358904011547565460205078125;-0.01180833391845226287841796875;-0.011808327399194240570068359375;0.0034835883416235446929931640625;0.3332020342350006103515625;-0.0034835846163332462310791015625;0.3332020342350006103515625;-0.333202064037322998046875;-0.003483586013317108154296875]
      mask Display: e = 0.06;c1 = [120 150 230]/255;c2 = ([120 150 230]+0)/383;c3 = ([120 150 230]+128)/383;patch([0 1 1 0],[0 0 1 1],c1);patch([0 1 1 1-e 1-e 0+e],[0 0 1 1-e 0+e 0+e],c2);patch([0 0 1 1-e 0+e 0+e],[0 1 1 1-e 1-e 0+e],c3);plot([0 1 1 0 0],[0 0 1 1 0]);disp('weights');
  "IW{2,1}(9,:)'" : Constant  Value=[0.333259999752044677734375;-0.00046248571015894412994384765625;-0.00044886427349410951137542724609375;-0.3332599699497222900390625;-0.00921399891376495361328125;-0.333262860774993896484375;0.333259999752044677734375;-0.009829509072005748748779296875;0.333259999752044677734375;0.009213999845087528228759765625;-0.333260595798492431640625;0.0004624905996024608612060546875;-0.00921400450170040130615234375;-0.00921399705111980438232421875;-0.00046247732825577259063720703125;0.333259999752044677734375;0.00046247430145740509033203125;0.333259999752044677734375;-0.333259999752044677734375;0.000462484429590404033660888671875]
      mask Display: e = 0.06;c1 = [120 150 230]/255;c2 = ([120 150 230]+0)/383;c3 = ([120 150 230]+128)/383;patch([0 1 1 0],[0 0 1 1],c1);patch([0 1 1 1-e 1-e 0+e],[0 0 1 1-e 0+e 0+e],c2);patch([0 0 1 1-e 0+e 0+e],[0 1 1 1-e 1-e 0+e],c3);plot([0 1 1 0 0],[0 0 1 1 0]);disp('weights');
  Mux : Mux  Inputs=20
      mask Display: e = 0.06;c1 = [120 150 230]/255;c2 = ([120 150 230]+0)/383;c3 = ([120 150 230]+128)/383;patch([0 1 1 0],[0 0 1 1],c1);patch([0 1 1 1-e 1-e 0+e],[0 0 1 1-e 0+e 0+e],c2);patch([0 0 1 1-e 0+e 0+e],[0 1 1 1-e 1-e 0+e],c3);plot([0 1 1 0 0],[0 0 1 1 0]);disp('Mux');
  dotprod{1..20} (20 alike) : neural/Weight Functions/dotprod
  "lz{2,1}" : Outport
      mask Display: e = 0.06;c1 = [120 230 180]/255;c2 = ([120 230 180]+0)/(256+128);c3 = ([120 230 180]+128)/(256+128);patch([0 1 1 0],[0 0 1 1],c1);patch([0 1 1 1-e 1-e 0+e],[0 0 1 1-e 0+e 0+e],c2);patch([0 0 1 1-e 0+e 0+e],[0 1 1 1-e 1-e 0+e],c3);plot([0 1 1 0 0],[0 0 1 1 0]);
  wires:
  Mux/1 -> "lz{2,1}"/1
  dotprod20/1 -> Mux/20
  "IW{2,1}(20,:)'"/1 -> dotprod20/1
  dotprod19/1 -> Mux/19
  "IW{2,1}(19,:)'"/1 -> dotprod19/1
  dotprod18/1 -> Mux/18
  "IW{2,1}(18,:)'"/1 -> dotprod18/1
  dotprod17/1 -> Mux/17
  "IW{2,1}(17,:)'"/1 -> dotprod17/1
  dotprod16/1 -> Mux/16
  "IW{2,1}(16,:)'"/1 -> dotprod16/1
  dotprod15/1 -> Mux/15
  "IW{2,1}(15,:)'"/1 -> dotprod15/1
  dotprod14/1 -> Mux/14
  "IW{2,1}(14,:)'"/1 -> dotprod14/1
  dotprod13/1 -> Mux/13
  "IW{2,1}(13,:)'"/1 -> dotprod13/1
  dotprod12/1 -> Mux/12
  "IW{2,1}(12,:)'"/1 -> dotprod12/1
  dotprod11/1 -> Mux/11
  "IW{2,1}(11,:)'"/1 -> dotprod11/1
  dotprod10/1 -> Mux/10
  "IW{2,1}(10,:)'"/1 -> dotprod10/1
  dotprod9/1 -> Mux/9
  "IW{2,1}(9,:)'"/1 -> dotprod9/1
  dotprod8/1 -> Mux/8
  "IW{2,1}(8,:)'"/1 -> dotprod8/1
  dotprod7/1 -> Mux/7
  "IW{2,1}(7,:)'"/1 -> dotprod7/1
  dotprod6/1 -> Mux/6
  "IW{2,1}(6,:)'"/1 -> dotprod6/1
  dotprod5/1 -> Mux/5
  "IW{2,1}(5,:)'"/1 -> dotprod5/1
  dotprod4/1 -> Mux/4
  "IW{2,1}(4,:)'"/1 -> dotprod4/1
  dotprod3/1 -> Mux/3
  "IW{2,1}(3,:)'"/1 -> dotprod3/1
  dotprod2/1 -> Mux/2
  "IW{2,1}(2,:)'"/1 -> dotprod2/1
  dotprod1/1 -> Mux/1
  "ad{2,1}"/1 -> dotprod20/2, dotprod19/2, dotprod18/2, dotprod17/2, dotprod16/2, dotprod15/2, dotprod14/2, dotprod13/2, dotprod12/2, dotprod11/2, dotprod10/2, dotprod9/2, dotprod8/2, dotprod7/2, dotprod6/2, dotprod5/2, dotprod4/2, dotprod3/2, dotprod2/2, dotprod1/2
  "IW{2,1}(1,:)'"/1 -> dotprod1/1

== system MPC_stateflow/Verisig Controller 2/Layer 3/Delays 1 ==
  "p{3}" : Inport  PortDimensions=20
      mask Display: e = 0.06;c1 = [120 230 180]/255;c2 = ([120 230 180]+0)/(256+128);c3 = ([120 230 180]+128)/(256+128);patch([0 1 1 0],[0 0 1 1],c1);patch([0 1 1 1-e 1-e 0+e],[0 0 1 1-e 0+e 0+e],c2);patch([0 0 1 1-e 0+e 0+e],[0 1 1 1-e 1-e 0+e],c3);plot([0 1 1 0 0],[0 0 1 1 0]);
  mux : Mux  Inputs=1
      mask Display: e = 0.06;c1 = [120 150 230]/255;c2 = ([120 150 230]+0)/383;c3 = ([120 150 230]+128)/383;patch([0 1 1 0],[0 0 1 1],c1);patch([0 1 1 1-e 1-e 0+e],[0 0 1 1-e 0+e 0+e],c2);patch([0 0 1 1-e 0+e 0+e],[0 1 1 1-e 1-e 0+e],c3);plot([0 1 1 0 0],[0 0 1 1 0]);disp('Mux')
  "pd{3,2}" : Outport
      mask Display: e = 0.06;c1 = [120 230 180]/255;c2 = ([120 230 180]+0)/(256+128);c3 = ([120 230 180]+128)/(256+128);patch([0 1 1 0],[0 0 1 1],c1);patch([0 1 1 1-e 1-e 0+e],[0 0 1 1-e 0+e 0+e],c2);patch([0 0 1 1-e 0+e 0+e],[0 1 1 1-e 1-e 0+e],c3);plot([0 1 1 0 0],[0 0 1 1 0]);
  wires:
  mux/1 -> "pd{3,2}"/1
  "p{3}"/1 -> mux/1

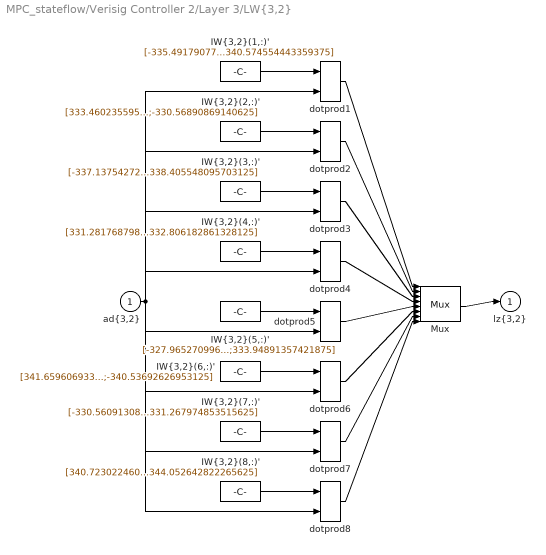
== system MPC_stateflow/Verisig Controller 2/Layer 3/LW{3,2} ==
  "ad{3,2}" : Inport  PortDimensions=20
      mask Display: e = 0.06;c1 = [120 230 180]/255;c2 = ([120 230 180]+0)/(256+128);c3 = ([120 230 180]+128)/(256+128);patch([0 1 1 0],[0 0 1 1],c1);patch([0 1 1 1-e 1-e 0+e],[0 0 1 1-e 0+e 0+e],c2);patch([0 0 1 1-e 0+e 0+e],[0 1 1 1-e 1-e 0+e],c3);plot([0 1 1 0 0],[0 0 1 1 0]);
  "IW{3,2}(1,:)'" : Constant  Value=[-335.491790771484375;295.449859619140625;-300.990753173828125;292.68359375;439.89520263671875;340.986480712890625;341.376861572265625;-446.518585205078125;-442.758331298828125;283.715728759765625;-300.080841064453125;-300.40203857421875;-298.267974853515625;-338.424774169921875;-298.95599365234375;342.16082763671875;-442.63568115234375;340.798248291015625;291.43646240234375;340.574554443359375]
      mask Display: e = 0.06;c1 = [120 150 230]/255;c2 = ([120 150 230]+0)/383;c3 = ([120 150 230]+128)/383;patch([0 1 1 0],[0 0 1 1],c1);patch([0 1 1 1-e 1-e 0+e],[0 0 1 1-e 0+e 0+e],c2);patch([0 0 1 1-e 0+e 0+e],[0 1 1 1-e 1-e 0+e],c3);plot([0 1 1 0 0],[0 0 1 1 0]);disp('weights');
  "IW{3,2}(2,:)'" : Constant  Value=[333.460235595703125;283.688446044921875;-290.77532958984375;284.634857177734375;458.39697265625;-331.57843017578125;-330.1046142578125;-458.7938232421875;-459.342010498046875;277.321441650390625;-290.092193603515625;-291.56329345703125;-287.394195556640625;332.539215087890625;-289.87408447265625;-327.3385009765625;-456.78961181640625;-331.62420654296875;282.5384521484375;-330.56890869140625]
      mask Display: e = 0.06;c1 = [120 150 230]/255;c2 = ([120 150 230]+0)/383;c3 = ([120 150 230]+128)/383;patch([0 1 1 0],[0 0 1 1],c1);patch([0 1 1 1-e 1-e 0+e],[0 0 1 1-e 0+e 0+e],c2);patch([0 0 1 1-e 0+e 0+e],[0 1 1 1-e 1-e 0+e],c3);plot([0 1 1 0 0],[0 0 1 1 0]);disp('weights');
  "IW{3,2}(3,:)'" : Constant  Value=[-337.137542724609375;289.10272216796875;-294.45098876953125;296.287078857421875;-438.852508544921875;339.534088134765625;337.741485595703125;435.8607177734375;437.567138671875;293.135589599609375;-295.780120849609375;-293.802703857421875;-295.40887451171875;-337.87371826171875;-293.361175537109375;339.543914794921875;437.253631591796875;338.9185791015625;289.39752197265625;338.405548095703125]
      mask Display: e = 0.06;c1 = [120 150 230]/255;c2 = ([120 150 230]+0)/383;c3 = ([120 150 230]+128)/383;patch([0 1 1 0],[0 0 1 1],c1);patch([0 1 1 1-e 1-e 0+e],[0 0 1 1-e 0+e 0+e],c2);patch([0 0 1 1-e 0+e 0+e],[0 1 1 1-e 1-e 0+e],c3);plot([0 1 1 0 0],[0 0 1 1 0]);disp('weights');
  "IW{3,2}(4,:)'" : Constant  Value=[331.281768798828125;278.56243896484375;-286.856597900390625;290.38287353515625;-383.39654541015625;-332.671630859375;-332.413604736328125;458.237274169921875;394.3974609375;288.79791259765625;-287.97247314453125;-287.65728759765625;-287.882110595703125;333.19647216796875;-286.55657958984375;-330.171783447265625;458.907989501953125;-332.555511474609375;282.837860107421875;-332.806182861328125]
      mask Display: e = 0.06;c1 = [120 150 230]/255;c2 = ([120 150 230]+0)/383;c3 = ([120 150 230]+128)/383;patch([0 1 1 0],[0 0 1 1],c1);patch([0 1 1 1-e 1-e 0+e],[0 0 1 1-e 0+e 0+e],c2);patch([0 0 1 1-e 0+e 0+e],[0 1 1 1-e 1-e 0+e],c3);plot([0 1 1 0 0],[0 0 1 1 0]);disp('weights');
  "IW{3,2}(5,:)'" : Constant  Value=[-327.96527099609375;-282.675201416015625;281.63214111328125;-289.458892822265625;376.37738037109375;333.953521728515625;335.018402099609375;-457.103485107421875;-390.469696044921875;-294.422332763671875;281.446380615234375;281.694000244140625;284.767364501953125;-332.499725341796875;284.126861572265625;335.67401123046875;-454.148040771484375;334.2760009765625;-288.58868408203125;333.94891357421875]
      mask Display: e = 0.06;c1 = [120 150 230]/255;c2 = ([120 150 230]+0)/383;c3 = ([120 150 230]+128)/383;patch([0 1 1 0],[0 0 1 1],c1);patch([0 1 1 1-e 1-e 0+e],[0 0 1 1-e 0+e 0+e],c2);patch([0 0 1 1-e 0+e 0+e],[0 1 1 1-e 1-e 0+e],c3);plot([0 1 1 0 0],[0 0 1 1 0]);disp('weights');
  "IW{3,2}(6,:)'" : Constant  Value=[341.65960693359375;-295.740264892578125;292.73046875;-298.508575439453125;437.528228759765625;-340.933502197265625;-338.32208251953125;-443.305511474609375;-439.650604248046875;-301.749359130859375;292.287872314453125;291.448211669921875;295.3114013671875;341.15484619140625;294.27960205078125;-337.8680419921875;-440.09320068359375;-340.21820068359375;-298.207672119140625;-340.53692626953125]
      mask Display: e = 0.06;c1 = [120 150 230]/255;c2 = ([120 150 230]+0)/383;c3 = ([120 150 230]+128)/383;patch([0 1 1 0],[0 0 1 1],c1);patch([0 1 1 1-e 1-e 0+e],[0 0 1 1-e 0+e 0+e],c2);patch([0 0 1 1-e 0+e 0+e],[0 1 1 1-e 1-e 0+e],c3);plot([0 1 1 0 0],[0 0 1 1 0]);disp('weights');
  "IW{3,2}(7,:)'" : Constant  Value=[-330.5609130859375;-291.566986083984375;287.873077392578125;-286.07989501953125;-456.10418701171875;332.381011962890625;332.67425537109375;451.767852783203125;455.01104736328125;-287.474090576171875;285.10052490234375;287.636810302734375;286.707672119140625;-332.678009033203125;289.909942626953125;333.337554931640625;453.990264892578125;332.972076416015625;-292.476287841796875;331.267974853515625]
      mask Display: e = 0.06;c1 = [120 150 230]/255;c2 = ([120 150 230]+0)/383;c3 = ([120 150 230]+128)/383;patch([0 1 1 0],[0 0 1 1],c1);patch([0 1 1 1-e 1-e 0+e],[0 0 1 1-e 0+e 0+e],c2);patch([0 0 1 1-e 0+e 0+e],[0 1 1 1-e 1-e 0+e],c3);plot([0 1 1 0 0],[0 0 1 1 0]);disp('weights');
  "IW{3,2}(8,:)'" : Constant  Value=[340.7230224609375;-301.74951171875;296.970977783203125;-292.657196044921875;-440.14434814453125;-343.39404296875;-343.332305908203125;441.12506103515625;440.001007080078125;-290.798492431640625;294.84613037109375;295.703399658203125;296.45263671875;342.21826171875;298.08880615234375;-341.65997314453125;440.384613037109375;-343.41845703125;-299.17828369140625;-344.052642822265625]
      mask Display: e = 0.06;c1 = [120 150 230]/255;c2 = ([120 150 230]+0)/383;c3 = ([120 150 230]+128)/383;patch([0 1 1 0],[0 0 1 1],c1);patch([0 1 1 1-e 1-e 0+e],[0 0 1 1-e 0+e 0+e],c2);patch([0 0 1 1-e 0+e 0+e],[0 1 1 1-e 1-e 0+e],c3);plot([0 1 1 0 0],[0 0 1 1 0]);disp('weights');
  Mux : Mux  Inputs=8
      mask Display: e = 0.06;c1 = [120 150 230]/255;c2 = ([120 150 230]+0)/383;c3 = ([120 150 230]+128)/383;patch([0 1 1 0],[0 0 1 1],c1);patch([0 1 1 1-e 1-e 0+e],[0 0 1 1-e 0+e 0+e],c2);patch([0 0 1 1-e 0+e 0+e],[0 1 1 1-e 1-e 0+e],c3);plot([0 1 1 0 0],[0 0 1 1 0]);disp('Mux');
  dotprod{1..8} (8 alike) : neural/Weight Functions/dotprod
  "lz{3,2}" : Outport
      mask Display: e = 0.06;c1 = [120 230 180]/255;c2 = ([120 230 180]+0)/(256+128);c3 = ([120 230 180]+128)/(256+128);patch([0 1 1 0],[0 0 1 1],c1);patch([0 1 1 1-e 1-e 0+e],[0 0 1 1-e 0+e 0+e],c2);patch([0 0 1 1-e 0+e 0+e],[0 1 1 1-e 1-e 0+e],c3);plot([0 1 1 0 0],[0 0 1 1 0]);
  wires:
  Mux/1 -> "lz{3,2}"/1
  dotprod8/1 -> Mux/8
  "IW{3,2}(8,:)'"/1 -> dotprod8/1
  dotprod7/1 -> Mux/7
  "IW{3,2}(7,:)'"/1 -> dotprod7/1
  dotprod6/1 -> Mux/6
  "IW{3,2}(6,:)'"/1 -> dotprod6/1
  dotprod5/1 -> Mux/5
  "IW{3,2}(5,:)'"/1 -> dotprod5/1
  dotprod4/1 -> Mux/4
  "IW{3,2}(4,:)'"/1 -> dotprod4/1
  dotprod3/1 -> Mux/3
  "IW{3,2}(3,:)'"/1 -> dotprod3/1
  dotprod2/1 -> Mux/2
  "IW{3,2}(2,:)'"/1 -> dotprod2/1
  dotprod1/1 -> Mux/1
  "ad{3,2}"/1 -> dotprod8/2, dotprod7/2, dotprod6/2, dotprod5/2, dotprod4/2, dotprod3/2, dotprod2/2, dotprod1/2
  "IW{3,2}(1,:)'"/1 -> dotprod1/1

== stateflow chart MPC_stateflow/Quadrotor and planner ==
  settings: updateMethod=CONTINUOUS  sampleTime=0.1
  state Following
    du:
    bx_dot = 0.25;
    by_dot = -0.25
    bz_dot = 0.25;
    px_dot = vx;
    py_dot = vy;
    pz_dot = vz;
    vx_dot = 9.81 * tan(pitch);
    vy_dot = -9.81 * tan(roll);
    vz_dot = thrust - 9.81;
    %Outputs
    px_out = px-bx;
    py_out = py-by;
    pz_out = pz-bz;
    vx_out = vx;
    vy_out = vy;
    vz_out = vz;
    bx_out = bx;
    by_out = by;
    bz_out = bz;
  (default) -> Following : {px = 0.15;
      | py = 0.15;
      | pz = 0.1;
      | vx = 0;
      | vy = 0;
      | vz = 0;
      | bx = 0.2;
      | by = 0.1;
      | bz = 0.1;}
  data: px local; py local; pz local; vx local; px_out output; py_out output; pz_out output; vx_out output; pitch input; roll input; thrust input; vy local; vz local; vy_out output; vz_out output; bx local; by local; bz local; bx_out output; by_out output; bz_out output
  data px settings: updateMethod=SF_CONTINUOUS_TIME_DATA
  data py settings: updateMethod=SF_CONTINUOUS_TIME_DATA
  data pz settings: updateMethod=SF_CONTINUOUS_TIME_DATA
  data vx settings: updateMethod=SF_CONTINUOUS_TIME_DATA
  data vy settings: updateMethod=SF_CONTINUOUS_TIME_DATA
  data vz settings: updateMethod=SF_CONTINUOUS_TIME_DATA
  data bx settings: updateMethod=SF_CONTINUOUS_TIME_DATA
  data by settings: updateMethod=SF_CONTINUOUS_TIME_DATA
  data bz settings: updateMethod=SF_CONTINUOUS_TIME_DATA

== matlab function MPC_stateflow/MATLAB Function ==
  data: u input; y output
function y = fcn(u)

if u(1) == max(u)
    x = [-0.1;-0.1;7.81];
elseif u(2) == max(u)
    x = [-0.1;-0.1;11.81];
elseif u(3) == max(u)
    x = [-0.1;0.1;7.81];
elseif u(4) == max(u)
    x = [-0.1;0.1;11.81];
elseif u(5) == max(u)
    x = [0.1;-0.1;7.81];
elseif u(6) == max(u)
    x = [0.1;-0.1;11.81];
elseif u(7) == max(u)
    x = [0.1;0.1;7.81];
else
    x = [0.1;0.1;11.81];
end

y = x;

== matlab function MPC_stateflow/MATLAB Function1 ==
  data: u input; y output
function y = fcn(u)

if u(1) == max(u)
    x = [-0.1;-0.1;7.81];
elseif u(2) == max(u)
    x = [-0.1;-0.1;11.81];
elseif u(3) == max(u)
    x = [-0.1;0.1;7.81];
elseif u(4) == max(u)
    x = [-0.1;0.1;11.81];
elseif u(5) == max(u)
    x = [0.1;-0.1;7.81];
elseif u(6) == max(u)
    x = [0.1;-0.1;11.81];
elseif u(7) == max(u)
    x = [0.1;0.1;7.81];
else
    x = [0.1;0.1;11.81];
end

y = x;

== stateflow chart MPC_stateflow/Quadrotor and planner1 ==
  settings: updateMethod=CONTINUOUS  sampleTime=0.1
  state Following
    du:
    bx_dot = 0.25;
    by_dot = -0.25;
    bz_dot = 0.25;
    px_dot = vx;
    py_dot = vy;
    pz_dot = vz;
    vx_dot = 9.81 * tan(pitch);
    vy_dot = -9.81 * tan(roll);
    vz_dot = thrust - 9.81;
    %Outputs
    px_out = px-bx;
    py_out = py-by;
    pz_out = pz-bz;
    vx_out = vx;
    vy_out = vy;
    vz_out = vz;
    bx_out = bx;
    by_out = by;
    bz_out = bz;
  (default) -> Following : {px = 0.15;
      | py = 0.15;
      | pz = 0.1;
      | vx = 0;
      | vy = 0;
      | vz = 0;
      | bx = 0.2;
      | by = 0.1;
      | bz = 0.1;}
  data: px local; py local; pz local; vx local; px_out output; py_out output; pz_out output; vx_out output; pitch input; roll input; thrust input; vy local; vz local; vy_out output; vz_out output; bx local; by local; bz local; bx_out output; by_out output; bz_out output
  data px settings: updateMethod=SF_CONTINUOUS_TIME_DATA
  data py settings: updateMethod=SF_CONTINUOUS_TIME_DATA
  data pz settings: updateMethod=SF_CONTINUOUS_TIME_DATA
  data vx settings: updateMethod=SF_CONTINUOUS_TIME_DATA
  data vy settings: updateMethod=SF_CONTINUOUS_TIME_DATA
  data vz settings: updateMethod=SF_CONTINUOUS_TIME_DATA
  data bx settings: updateMethod=SF_CONTINUOUS_TIME_DATA
  data by settings: updateMethod=SF_CONTINUOUS_TIME_DATA
  data bz settings: updateMethod=SF_CONTINUOUS_TIME_DATA
